simulink model "cps_blockB_camera_v2"  (R2012b)
settings: Solver=FixedStepDiscrete  StartTime=0.0  StopTime=8.5  RelTol=20e-5
model workspace (MAT data in the model file):
  ini_nozzle_vpos = 0.3
  ini_B_block_vpos = 0.01
  ini_G_block_vpos = 0.11
  block_height = 0.3
libraries: vrlib x1, cps_lib_v2 x1
settings Model: Creator=pmosterm  LastModifiedBy=pmosterm
settings SolverCC: ZcThreshold=2e-5  MaxConsecutiveZCs=20  EnableConcurrentExecution=on  ConcurrentTasks=on  ZeroCrossAlgorithm=Adaptive  SolverResetMethod=Robust
settings OptimizationCC: InlineParams=on
settings DebuggingCC: ReadBeforeWriteMsg=DisableAll  WriteAfterWriteMsg=DisableAll  WriteAfterReadMsg=DisableAll  AlgebraicLoopMsg=error  UnderspecifiedInitializationDetection=Simplified  FcnCallInpInsideContextMsg=EnableAllAsWarning  ModelReferenceExtraNoncontSigs=warning
settings GRTTargetCC: CombineOutputUpdateFcns=off  GRTInterface=on
settings ConfigurationSet: Description=SimMechanics 2G

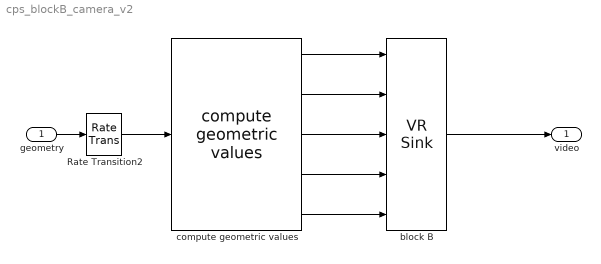
== system cps_blockB_camera_v2 ==
  geometry : Inport  OutDataTypeStr=Bus: slBusGeometry  SampleTime=0.005
  Rate Transition2 : RateTransition  Deterministic=off  OutPortSampleTime=0.1
  block B : vrlib/VR Sink  InstantiateOnLoad=on  SampleTime=0.1  ViewEnable=on  RemoteChange=off  RemoteView=off  FieldsWritten=red_block2x3dim.translation.3.1.1.double#slider.translation.3.1.1.double#LOWER.translation.3.1.1.double#purple_block2x3dim.translation.3.1.1.double#blue_block2x3dim.translation.3.1.1.double  WorldFileName=cps_world_v2.wrl  AutoView=off  VideoDimensions=[240 120]  AllowVariableSize=off  FigureProperties="{'Position', 'Name', 'Viewpoint', 'CameraBound', 'CameraDirection', 'CameraPosition', 'CameraUpVector', 'ZoomFactor', 'Antialiasing', 'Headlight', 'Lighting', 'NavPanel', 'StatusBar', 'ToolBar', 'Textures', 'Transparency', 'Triad', 'Wireframe', 'NavZones', 'NavMode', 'NavSpeed', 'CaptureFileFormat', 'CaptureFileName', 'Record2DCompressMethod', 'Record2DCompressQuality', 'Record2D', 'Record2DFileName', 'Record2DFPS'; [5.2000000000000000e+02   6.0000000000000000e+01   1.2000000000000000e+02   2.4000000000000000e+02], '', 'Block B viewpoint', 'on', [0.0000000000000000e+00   0.0000000000000000e+00  -1.0000000000000000e+00], [0.0000000000000000e+00   0.0000000000000000e+00   0.0000000000000000e+00], [0.0000000000000000e+00   1.0000000000000000e+00   0.0000000000000000e+00], [1.0000000000000000e+00], 'on', 'on', 'on', 'none', 'off', 'off', 'on', 'on', 'none', 'off', 'off', 'walk', 'normal', 'tif', '%f_anim_%n.tif', 'auto', [7.5000000000000000e+01], 'off', '***video***', [1.5000000000000000e+01]}"
  compute geometric values : cps_lib_v2/compute geometric values
  video : Outport
  wires:
  block B/1 -> video/1
  geometry/1 -> Rate Transition2/1
  compute geometric values/3 -> block B/3
  compute geometric values/2 -> block B/2
  compute geometric values/4 -> block B/4
  compute geometric values/1 -> block B/1
  compute geometric values/5 -> block B/5
  Rate Transition2/1 -> compute geometric values/1
